simulink model "problem3"  (R2024b)
settings: Solver=VariableStepAuto  StartTime=0.0  StopTime=100  RelTol=1e-3
values from neighbouring files (symbols this model uses):
  alpha_1 = 0.0952    [problem3.m]    (also in problem3_constants.m; problem3_setup.m)
  beta_1 = -0.9048    [problem3.m]    (also in problem3_constants.m; problem3_setup.m)
settings Model: Creator=djd14  LastModifiedBy=djd14

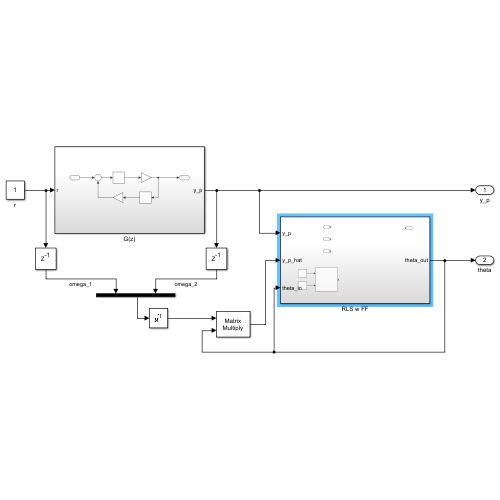
[thumbnail: Simulink's stored preview of the top-level diagram]
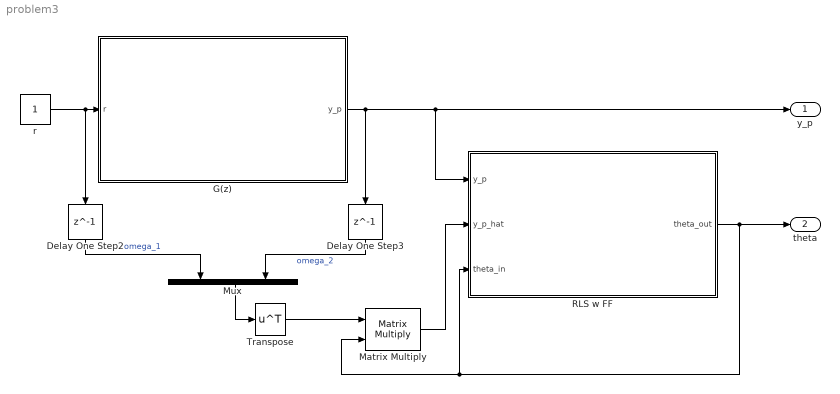
== system problem3 ==
  Delay One Step2 : Delay  DelayLength=1
  Delay One Step3 : Delay  DelayLength=1
  G(z) : Subsystem
  Matrix Multiply : Product  Multiplication=Matrix(*)
  Mux : Mux  Inputs=2
  RLS w FF : Subsystem
  Transpose : Math  Operator=transpose
  r : Constant
  y_p : Outport
  theta : Outport  Port=2
  wires:
  r/1 -> G(z)/1(r), Delay One Step2/1
  Delay One Step2/1 -> Mux/1  "omega_1"
  Delay One Step3/1 -> Mux/2  "omega_2"
  Mux/1 -> Transpose/1
  Transpose/1 -> Matrix Multiply/1
  G(z)/1(y_p) -> RLS w FF/1(y_p), y_p/1, Delay One Step3/1
  RLS w FF/1(theta_out) -> theta/1, RLS w FF/3(theta_in), Matrix Multiply/2
  Matrix Multiply/1 -> RLS w FF/2(y_p_hat)

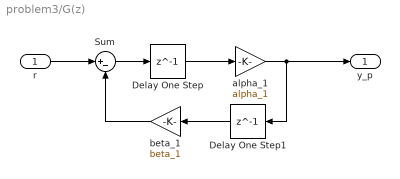
== system problem3/G(z) ==
  r : Inport
  Delay One Step : Delay  DelayLength=1
  Delay One Step1 : Delay  DelayLength=1
  Sum : Sum  Inputs=|+-
  alpha_1 : Gain  Gain=alpha_1
  beta_1 : Gain  Gain=beta_1
  y_p : Outport
  wires:
  alpha_1/1 -> y_p/1, Delay One Step1/1
  Sum/1 -> Delay One Step/1
  Delay One Step/1 -> alpha_1/1
  r/1 -> Sum/1
  beta_1/1 -> Sum/2
  Delay One Step1/1 -> beta_1/1

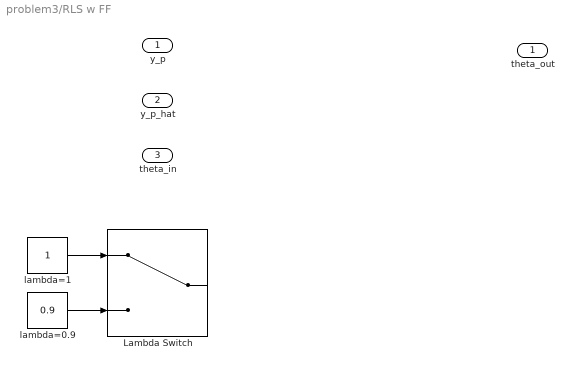
== system problem3/RLS w FF ==
  y_p : Inport
  y_p_hat : Inport  Port=2
  theta_in : Inport  Port=3
  Lambda Switch : ManualSwitch
  lambda=0.9 : Constant  Value=0.9
  lambda=1 : Constant
  theta_out : Outport
  wires:
  lambda=1/1 -> Lambda Switch/1
  lambda=0.9/1 -> Lambda Switch/2
